simulink model "DueSerbatoiPro"  (R2022b)
settings: Solver=VariableStepAuto  StartTime=0.0  StopTime=1000  RelTol=1e-3
values from neighbouring files (symbols this model uses):
  C1 = 10    [DueSerbatoiPro_values.m]
  C2 = 10    [DueSerbatoiPro_values.m]
  g = 9.81    [DueSerbatoiPro_values.m]
  Pa = 0    [DueSerbatoiPro_values.m]
  Q11 = 1    [DueSerbatoiPro_values.m]
  Q12 = 2    [DueSerbatoiPro_values.m]
  Q21 = 1    [DueSerbatoiPro_values.m]
  Q22 = 3    [DueSerbatoiPro_values.m]
  R1 = 1    [DueSerbatoiPro_values.m]
  R2 = 1    [DueSerbatoiPro_values.m]
  ro = 1000    [DueSerbatoiPro_values.m]
settings Model: Creator=giuli  LastModifiedBy=giuli

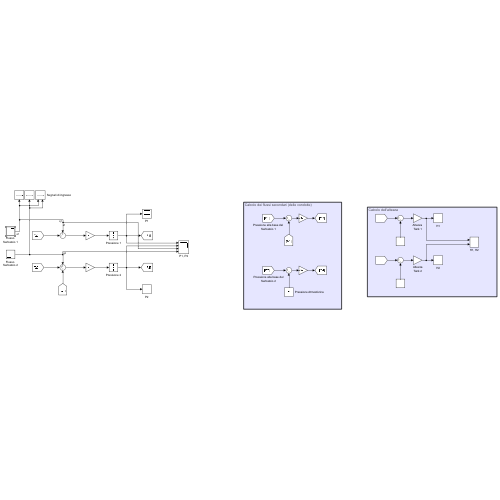
[thumbnail: Simulink's stored preview of the top-level diagram]
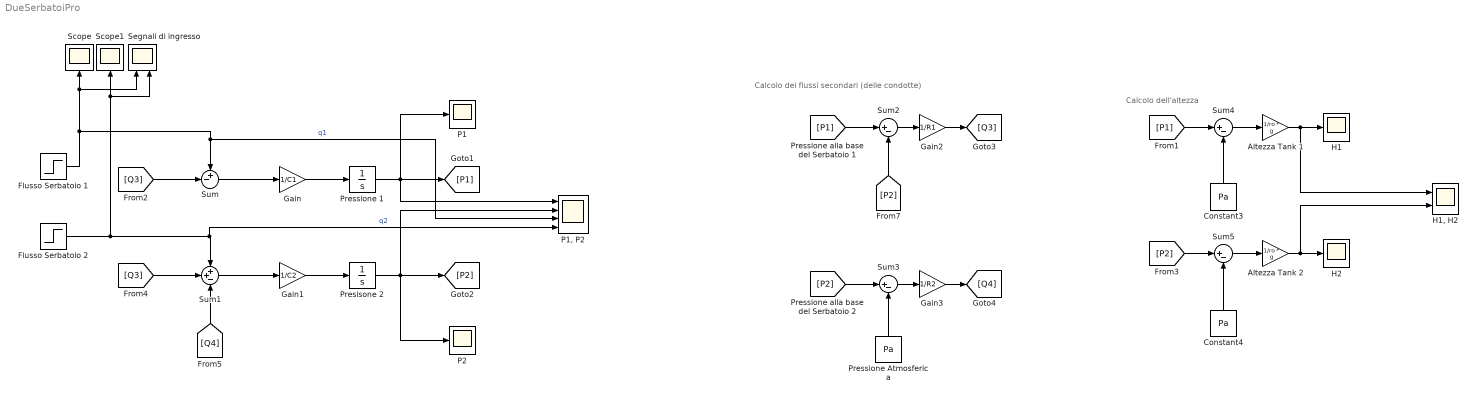
== system DueSerbatoiPro ==
  note: Calcolo dei flussi secondari (delle condotte)
  note: Calcolo dell'altezza
  Altezza Tank 2 : Gain  Gain=1/ro * g
  Altezza Tank 1 : Gain  Gain=1/ro * g
  Constant3 : Constant  Value=Pa
  Constant4 : Constant  Value=Pa
  Flusso Serbatoio 1 : Step  Time=500  Before=Q11  After=Q12  SampleTime=0.01
  Flusso Serbatoio 2 : Step  Time=800  Before=Q21  After=Q22  SampleTime=0.01
  Gain : Gain  Gain=1/C1
  Gain1 : Gain  Gain=1/C2
  Gain2 : Gain  Gain=1/R1
  Gain3 : Gain  Gain=1/R2
  H1 : Scope
  "H1, H2" : Scope  NumInputPorts=2
  H2 : Scope
  P1 : Scope
  "P1, P2" : Scope  NumInputPorts=4
  P2 : Scope
  Presisone 2 : Integrator
  Pressione 1 : Integrator
  Pressione Atmosferica : Constant  Value=Pa
  Scope : Scope
  Scope1 : Scope
  Segnali di ingresso : Scope  NumInputPorts=2
  Sum : Sum  Inputs=+-|
  Sum1 : Sum  Inputs=++-
  Sum{2..5} (4 alike) : Sum  Inputs=|+-
  wires:
  Pressione 1/1 -> "P1, P2"/1, [P1], P1/1
  Gain/1 -> Pressione 1/1
  Sum/1 -> Gain/1
  [Q3] -> Sum/2
  Gain1/1 -> Presisone 2/1
  Sum1/1 -> Gain1/1
  [Q3] -> Sum1/2
  [Q4] -> Sum1/3
  [P1] -> Sum2/1
  [P2] -> Sum2/2
  Sum2/1 -> Gain2/1
  Gain2/1 -> [Q3]
  Gain3/1 -> [Q4]
  Sum3/1 -> Gain3/1
  Pressione Atmosferica/1 -> Sum3/2
  [P2] -> Sum3/1
  Presisone 2/1 -> [P2], "P1, P2"/2, P2/1
  Constant3/1 -> Sum4/2
  [P1] -> Sum4/1
  Sum4/1 -> Altezza Tank 1/1
  Altezza Tank 1/1 -> "H1, H2"/1, H1/1
  Altezza Tank 2/1 -> "H1, H2"/2, H2/1
  Sum5/1 -> Altezza Tank 2/1
  [P2] -> Sum5/1
  Constant4/1 -> Sum5/2
  Flusso Serbatoio 2/1 -> Segnali di ingresso/2, Scope1/1, "P1, P2"/4, Sum1/1  "q2"
  Flusso Serbatoio 1/1 -> Segnali di ingresso/1, Scope/1, "P1, P2"/3, Sum/1  "q1"
